simulink model "test_GHV_open_smc"  (R2023b)
settings: Solver=FixedStepAuto  StartTime=0  StopTime=490  FixedStep=0.01  MaxStep=0.001  RelTol=1e-3
InitFcn:
  | run("init.m");
  | %load('feature_point_control_parameters.mat','feature_point_control_parameters');
model workspace (MAT data in the model file):
  initPosLLA = [0; 0; 30000]
undefined symbols (not defined in the file or in its folder): alpha_d_sample, GHV_cfg, t_sample
libraries: simulink_extras x6, aerolibasang x3, aerolibtransform2 x2, aerolib6dof2 x1, aerolibatmos2 x1, matrix_library x1, aerolibgravity2 x1, rllib x1
settings Model: SimulationMode=accelerator  Creator=Admin  LastModifiedBy=Admin
settings SolverCC: AllowMultiTaskInputOutput=on  ZeroCrossControl=EnableAll  ZeroCrossAlgorithm=Adaptive  AutoInsertRateTranBlk=on
settings DataIOCC: Refine=5
settings DebuggingCC: IgnoredZcDiagnostic=none

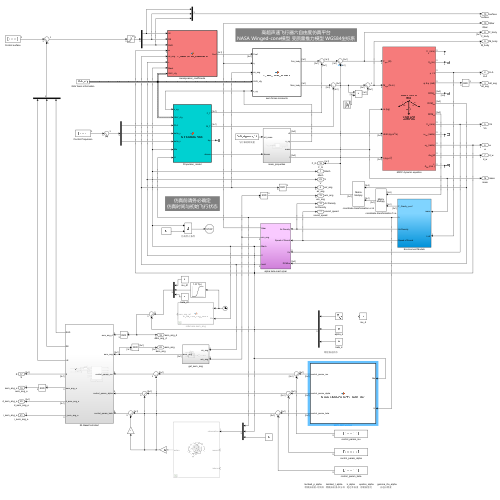
[thumbnail: Simulink's stored preview of the top-level diagram]
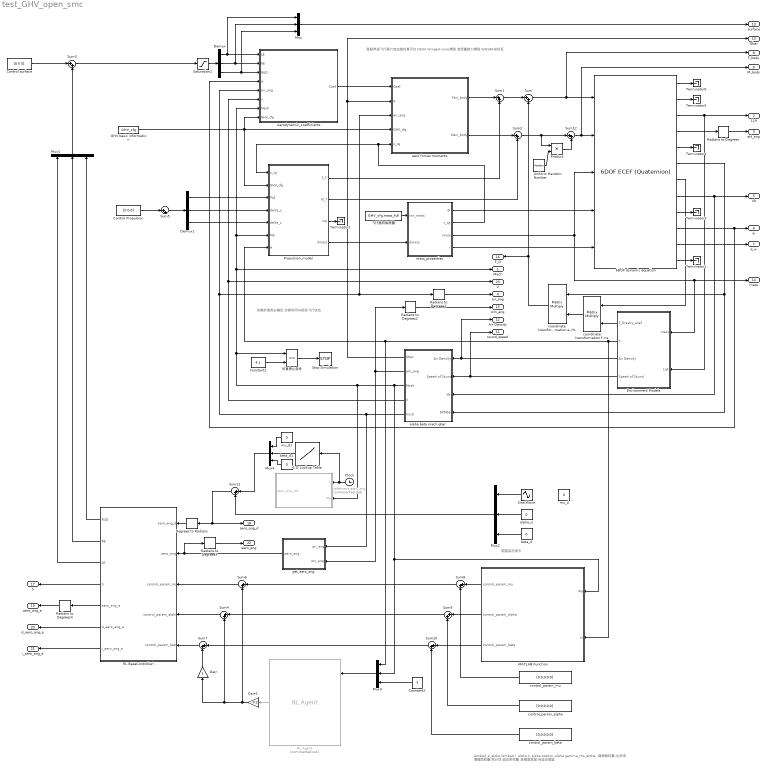
== system test_GHV_open_smc ==
  note: lambad_p_alpha       lambad_I_alpha       k_alpha       epsilon_alpha      gamma_rho_alpha
      | 增模面权重-比例项   增模面权重-积分项   趋近率权重   滑模面宽度             自适应增蓝
  note: 高超声速飞行器六自由度仿真平台
      | NASA Winged-cone模型 变质量推力模型 WGS84坐标系
  note: 仿真前请务必确定
      | 仿真时间与初始飞行状态
  note: 期望姿态指令
  1-D Lookup Table : Lookup_n-D  NumberOfTableDimensions=1  BreakpointsForDimension1=t_sample  Table=alpha_d_sample  InternalRulePriority=Speed  RndMeth=Simplest
  6DOF dynamic equation : aerolib6dof2/6DOF ECEF (Quaternion)  units=Metric (MKS)  mtype=Custom Variable  xg_0=LLA_init  Vm_0=Speed_init  eul_0=Euler_init  pm_0=Omega_init  mass_0=1.0  mass_e=0.5  mass_f=2.0  inertia=eye(3)  inertia_e=eye(3)  inertia_f=2*eye(3)  vre_flag=off  abi_flag=off  ptype=Custom  R=6378137  F=1/298.257223563  w_E=0  angle_in=Internal  LPM0=0  quat_statename=''  pm_statename=''  Vm_statename=''  posfixedframe_statename=''  posinertial_statename=''  LPM_statename=''  mass_statename=''
      settings: LibrarySourceBlock=|
      | aerolib6dof2/Custom Variable Mass 6DOF
      | ECEF (Quaternion)
  Aerodynamic_coefficients : MATLAB Function  TreatAsAtomicUnit=on
  Clock : Clock
  Constant1 : Constant  Value=4.1
  Constant2 : Constant  Value=5
  Control Propulsion : Constant  Value=[0 0 0]
  Control surface : Constant  Value=[0 0 0]
  Degrees to Radians : simulink_extras/Transformations/Degrees to Radians
  Demux : Demux  Outputs=3
  Demux1 : Demux  Outputs=3
  Environment Models : Subsystem
  GHV basic information : Constant  Value=GHV_cfg  VectorParams1D=off  OutDataTypeStr=Bus: slBus1
  Gain : Gain
  Gain1 : Gain  Gain=-0.2
  MATLAB Function : MATLAB Function  TreatAsAtomicUnit=on
  Mux{,1..4} (5 alike) : Mux  Inputs=3
  Product : Product
  Propulsion_model : MATLAB Function  TreatAsAtomicUnit=on
  RL Agent : rllib/RL Agent  Commented=on  Agent=agent_smc_RL_Trained_1  ExternalActionAsInput=off  ProvideLastAction=off  ProvideCumRwd=off  TreatAsDirectFeedthrough=on  UseStrictObservationDataTypes=off
  RL BaseControllerl : Subsystem
  Radians to Degrees{,1..4} (5 alike) : simulink_extras/Transformations/Radians to Degrees
  Saturation1 : Saturate  UpperLimit=30  LowerLimit=-30  ZeroCross=off
  Sine Wave : Sin  Amplitude=30  Frequency=0.05  SampleTime=0
  Stop Simulation : Stop
  Sum{,1..12} (13 alike) : Sum  Inputs=|++
  Terminator{1..6} (6 alike) : Terminator
  Uniform Random Number : UniformRandomNumber  Minimum=-0.1  Maximum=0.1  Seed=42  SampleTime=0.01
  aero forces moments : MATLAB Function  TreatAsAtomicUnit=on
  alpha beta mach qbar : Subsystem
  alpha_d : Constant  Value=0
  beta_d : Constant  Value=0
  beta_d1 : Constant  Value=0
  control_param_alpha : Constant  Value=[0;0;0;0;0]
  control_param_beta : Constant  Value=[0;0;0;0;0]
  control_param_mu : Constant  Value=[0;0;0;0;0]
  coordinate transformation e->b : Product  Multiplication=Matrix(*)
  coordinate transformation f->e : Product  Multiplication=Matrix(*)
  get_aero_ang : Subsystem
  mass_properties : Subsystem
  mu_d : Constant  Value=0
  mu_d1 : Constant  Value=0
  refernece aero_ang : MATLAB Function  Commented=on  TreatAsAtomicUnit=on
  仿真停止条件 : RelationalOperator  Operator=<=  OutDataTypeStr=boolean  RndMeth=Simplest  InputSameDT=off
  飞行器初始质量 : Constant  Value=GHV_cfg.mass_full
  Mach : Outport  SignalName=Mach
  LLA : Outport  Port=2  SignalName=LLA
  att_ang : Outport  Port=3  SignalName=att_ang
  air_ang : Outport  Port=4  SignalName=air_ang
  Vb : Outport  Port=5  SignalName=Vb
  w : Outport  Port=6  SignalName=w
  d_w : Outport  Port=7  SignalName=d_w
  F_body : Outport  Port=8  SignalName=F_body
  M_body : Outport  Port=9  SignalName=M_body
  Qbar : Outport  Port=10  SignalName=Qbar
  sound_speed : Outport  Port=11  SignalName=sound_speed
  Air Density : Outport  Port=12  SignalName=Air Density
  surface : Outport  Port=13  SignalName=surface
  mass : Outport  Port=14  SignalName=mass
  win_ang : Outport  Port=15  SignalName=win_ang
  F_G : Outport  Port=16  SignalName=F_G
  S : Outport  Port=17  SignalName=S
  aero_ang_d : Outport  Port=18  SignalName=aero_ang_d
  aero_ang_e : Outport  Port=19  SignalName=aero_ang_e
  d_aero_ang_e : Outport  Port=20  SignalName=d_aero_ang_e
  i_aero_ang_e : Outport  Port=21  SignalName=i_aero_ang_e
  aero_ang : Outport  Port=22  SignalName=aero_ang
  V : Outport  Port=23  SignalName=V
  wires:
  Control surface/1 -> Sum3/1
  coordinate transformation e->b/1 -> Sum/2, F_G/1
  Aerodynamic_coefficients/1(Coef) -> aero forces moments/1(Coef)
  mass_properties/2(x_cg) -> aero forces moments/5(x_cg), Propulsion_model/1(x_cg)
  coordinate transformation f->e/1 -> coordinate transformation e->b/2
  飞行器初始质量/1 -> mass_properties/1(init_mass)
  Radians to Degrees1/1 -> air_ang/1
  Propulsion_model/2(M_T) -> Sum2/2
  6DOF dynamic equation/1 -> Terminator6/1
  6DOF dynamic equation/9 -> Terminator3/1
  mass_properties/3(mass) -> 6DOF dynamic equation/3, Environment Models/1(mass), mass/1
  Radians to Degrees2/1 -> win_ang/1
  Demux/1 -> Aerodynamic_coefficients/1(LE), Mux/1
  6DOF dynamic equation/5 -> Terminator4/1
  Saturation1/1 -> Demux/1
  Demux1/2 -> Propulsion_model/4(delta_y)
  Control Propulsion/1 -> Sum5/1
  Propulsion_model/1(F_T) -> Sum1/2
  Demux/2 -> Aerodynamic_coefficients/2(RE), Mux/2
  alpha beta mach qbar/5(Incid) -> Aerodynamic_coefficients/5(air_ang), aero forces moments/3(air_ang), Radians to Degrees1/1, get_aero_ang/1(air_ang)
  Sum2/1 -> Sum12/1, Product/1
  Propulsion_model/4(dmass) -> mass_properties/2(dmass)
  Sum1/1 -> Sum/1
  Environment Models/3(Air Density) -> Air Density/1, alpha beta mach qbar/1(Air Density)
  Environment Models/2(h) -> Propulsion_model/7(H), Mux3/1, MATLAB Function/2(H)
  alpha beta mach qbar/1(Qbar) -> aero forces moments/2(q), Qbar/1
  aero forces moments/1(Fair_body) -> Sum1/1
  Radians to Degrees/1 -> att_ang/1
  aero forces moments/2(Mair_body) -> Sum2/1
  Demux1/3 -> Propulsion_model/5(delta_z)
  6DOF dynamic equation/10 -> w/1, Aerodynamic_coefficients/4(w)
  Mux/1 -> surface/1
  GHV basic information/1 -> aero forces moments/4(GHV_cfg), Propulsion_model/2(GHV_cfg), Aerodynamic_coefficients/8(GHV_cfg)
  Demux/3 -> Aerodynamic_coefficients/3(RUD), Mux/3
  alpha beta mach qbar/2(win_ang) -> Radians to Degrees2/1, get_aero_ang/2(win_ang)
  Sum3/1 -> Saturation1/1
  Propulsion_model/3(Isp) -> Terminator2/1
  Environment Models/1(F_Gravity_ecef) -> coordinate transformation f->e/2
  6DOF dynamic equation/11 -> d_w/1
  Demux1/1 -> Propulsion_model/3(PLA)
  mass_properties/1(dI) -> 6DOF dynamic equation/4
  6DOF dynamic equation/7 -> coordinate transformation f->e/1
  6DOF dynamic equation/2 -> Terminator5/1
  6DOF dynamic equation/8 -> Vb/1, alpha beta mach qbar/3(Vb)
  alpha beta mach qbar/4(V) -> Aerodynamic_coefficients/6(v), V/1
  Environment Models/4(Speed of Sound) -> sound_speed/1, alpha beta mach qbar/2(Speed of Sound)
  6DOF dynamic equation/12 -> Terminator1/1
  6DOF dynamic equation/4 -> Radians to Degrees/1
  Sum/1 -> 6DOF dynamic equation/1, F_body/1
  mass_properties/4(I) -> 6DOF dynamic equation/5
  Sum5/1 -> Demux1/1
  alpha beta mach qbar/3(Mach) -> Aerodynamic_coefficients/7(Mach), Propulsion_model/6(Ma), Mach/1, 仿真停止条件/1, refernece aero_ang/2(Ma), MATLAB Function/1(Ma), Mux3/2
  Constant1/1 -> 仿真停止条件/2
  仿真停止条件/1 -> Stop Simulation/1
  get_aero_ang/1(aero_ang) -> Radians to Degrees3/1, RL BaseControllerl/2(aero_ang)
  Sum11/1 -> Degrees to Radians/1, aero_ang_d/1
  RL BaseControllerl/1(RUD) -> Mux1/3
  RL BaseControllerl/2(RE) -> Mux1/2
  RL BaseControllerl/3(LE) -> Mux1/1
  RL BaseControllerl/4(S) -> S/1
  Degrees to Radians/1 -> RL BaseControllerl/1(aero_ang_d)
  Mux1/1 -> Sum3/2
  RL BaseControllerl/5(aero_ang_e) -> Radians to Degrees4/1
  RL BaseControllerl/6(d_aero_ang_e) -> d_aero_ang_e/1
  RL BaseControllerl/7(i_aero_ang_e) -> i_aero_ang_e/1
  6DOF dynamic equation/6 -> alpha beta mach qbar/4(DCMbe), coordinate transformation e->b/1
  6DOF dynamic equation/3 -> LLA/1, Environment Models/2(LLA)
  Sum6/1 -> RL BaseControllerl/3(control_param_mu)
  Radians to Degrees3/1 -> aero_ang/1
  Sum4/1 -> RL BaseControllerl/4(control_param_alpha)
  beta_d/1 -> Mux2/3
  alpha_d/1 -> Mux2/2
  Radians to Degrees4/1 -> aero_ang_e/1
  Mux3/1 -> RL Agent/1
  Constant2/1 -> Mux3/3
  Sum9/1 -> Sum4/1
  Sum8/1 -> Sum6/1
  RL Agent/1 -> Gain1/1
  Sum10/1 -> Sum7/1
  Gain/1 -> Sum7/2
  MATLAB Function/1(control_param_mu) -> Sum8/1
  MATLAB Function/2(control_param_alpha) -> Sum9/1
  MATLAB Function/3(control_param_beta) -> Sum10/1
  control_param_mu/1 -> Sum8/2
  control_param_alpha/1 -> Sum9/2
  control_param_beta/1 -> Sum10/2
  Clock/1 -> 1-D Lookup Table/1, refernece aero_ang/1(t)
  Mux2/1 -> Sum11/2
  Sum7/1 -> RL BaseControllerl/5(control_param_bate)
  Sine Wave/1 -> Mux2/1
  Gain1/1 -> Gain/1, Sum4/2, Sum6/2
  1-D Lookup Table/1 -> Mux4/2
  Mux4/1 -> Sum11/1
  mu_d1/1 -> Mux4/1
  beta_d1/1 -> Mux4/3
  Uniform Random Number/1 -> Product/2
  Sum12/1 -> M_body/1, 6DOF dynamic equation/2
  Product/1 -> Sum12/2

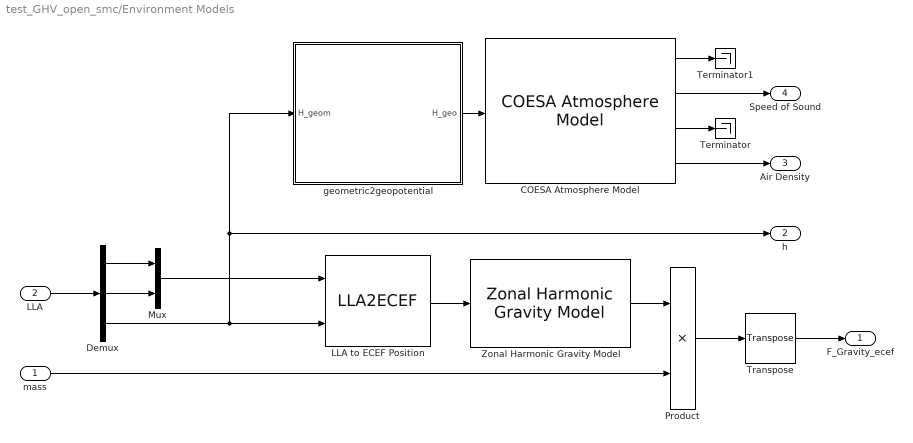
== system test_GHV_open_smc/Environment Models ==
  mass : Inport
  LLA : Inport  Port=2
  COESA Atmosphere Model : aerolibatmos2/COESA Atmosphere Model  units=Metric (MKS)  spec=1976 COESA-extended U.S. Standard Atmosphere  model=Profile  profile_var=High temperature  profile_percent=1%  profile_alt=5 km (16404 ft)  envelope_var=High temperature  envelope_percent=1%  action=Warning
  Demux : Demux  Outputs=3
  LLA to ECEF Position : LLA2ECEF
  Mux : Mux  Inputs=2
  Product : Product
  Terminator : Terminator
  Terminator1 : Terminator
  Transpose : matrix_library/Transpose
  Zonal Harmonic Gravity Model : aerolibgravity2/Zonal Harmonic Gravity Model  units=Metric (MKS)  degree=2  action=Warning  ptype=Earth  R=6378136.3  GM=398600441500000  jvalue=[1.0826269e-03 -2.5323000e-06 -1.6204000e-06]
  geometric2geopotential : MATLAB Function  TreatAsAtomicUnit=on
  F_Gravity_ecef : Outport
  h : Outport  Port=2
  Air Density : Outport  Port=3
  Speed of Sound : Outport  Port=4
  wires:
  COESA Atmosphere Model/1 -> Terminator1/1
  COESA Atmosphere Model/2 -> Speed of Sound/1
  COESA Atmosphere Model/3 -> Terminator/1
  COESA Atmosphere Model/4 -> Air Density/1
  LLA to ECEF Position/1 -> Zonal Harmonic Gravity Model/1
  Mux/1 -> LLA to ECEF Position/1
  Demux/3 -> h/1, geometric2geopotential/1(H_geom), LLA to ECEF Position/2
  Demux/1 -> Mux/1
  Demux/2 -> Mux/2
  LLA/1 -> Demux/1
  mass/1 -> Product/2
  Zonal Harmonic Gravity Model/1 -> Product/1
  Product/1 -> Transpose/1
  Transpose/1 -> F_Gravity_ecef/1
  geometric2geopotential/1(H_geo) -> COESA Atmosphere Model/1

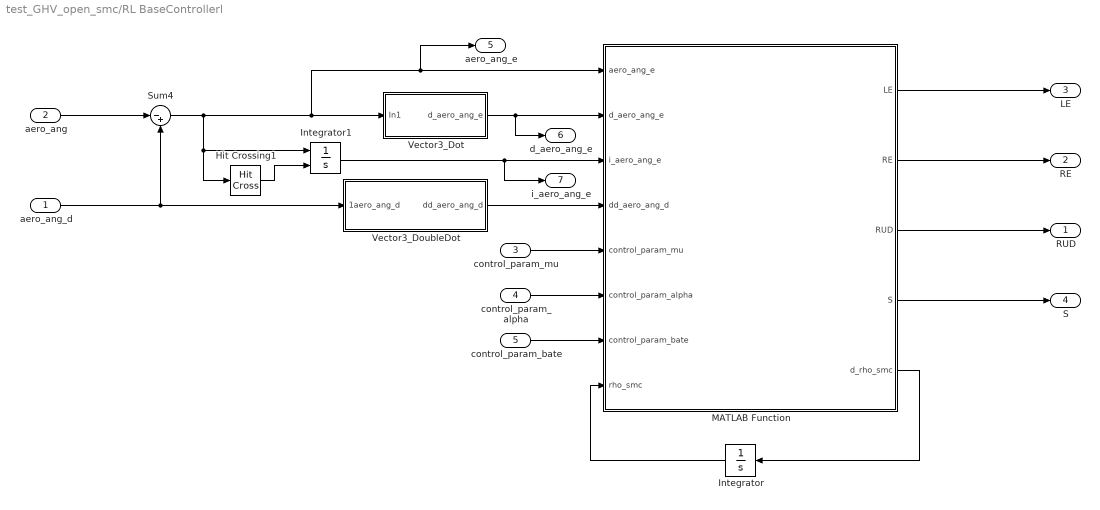
== system test_GHV_open_smc/RL BaseControllerl ==
  aero_ang_d : Inport
  aero_ang : Inport  Port=2
  control_param_mu : Inport  Port=3
  control_param_alpha : Inport  Port=4
  control_param_bate : Inport  Port=5
  Hit Crossing1 : HitCross
  Integrator : Integrator  InitialCondition=[0;10;0]
  Integrator1 : Integrator  ExternalReset=either
  MATLAB Function : MATLAB Function  TreatAsAtomicUnit=on
  Sum4 : Sum  Inputs=|-+
  Vector3_Dot : Subsystem
  Vector3_DoubleDot : Subsystem
  RUD : Outport
  RE : Outport  Port=2
  LE : Outport  Port=3
  S : Outport  Port=4
  aero_ang_e : Outport  Port=5
  d_aero_ang_e : Outport  Port=6
  i_aero_ang_e : Outport  Port=7
  wires:
  control_param_alpha/1 -> MATLAB Function/6(control_param_alpha)
  Vector3_DoubleDot/1(dd_aero_ang_d) -> MATLAB Function/4(dd_aero_ang_d)
  MATLAB Function/5(d_rho_smc) -> Integrator/1
  MATLAB Function/2(RE) -> RE/1
  aero_ang_d/1 -> Sum4/2, Vector3_DoubleDot/1(1aero_ang_d)
  MATLAB Function/1(LE) -> LE/1
  Integrator1/1 -> MATLAB Function/3(i_aero_ang_e), i_aero_ang_e/1
  MATLAB Function/3(RUD) -> RUD/1
  MATLAB Function/4(S) -> S/1
  Integrator/1 -> MATLAB Function/8(rho_smc)
  Sum4/1 -> Hit Crossing1/1, Integrator1/1, aero_ang_e/1, MATLAB Function/1(aero_ang_e), Vector3_Dot/1(In1)
  aero_ang/1 -> Sum4/1
  Hit Crossing1/1 -> Integrator1/2
  Vector3_Dot/1(d_aero_ang_e) -> MATLAB Function/2(d_aero_ang_e), d_aero_ang_e/1
  control_param_bate/1 -> MATLAB Function/7(control_param_bate)
  control_param_mu/1 -> MATLAB Function/5(control_param_mu)

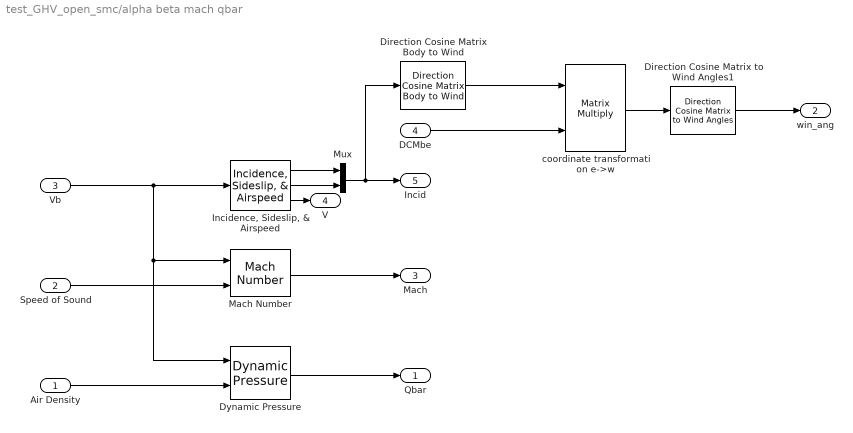
== system test_GHV_open_smc/alpha beta mach qbar ==
  Air Density : Inport
  Speed of Sound : Inport  Port=2
  Vb : Inport  Port=3
  DCMbe : Inport  Port=4
  Direction Cosine Matrix Body to Wind : aerolibtransform2/Direction Cosine Matrix Body to Wind
  Direction Cosine Matrix to Wind Angles1 : aerolibtransform2/Direction Cosine Matrix to Wind Angles  action=None  tolerance=eps(2)
  Dynamic Pressure : aerolibasang/Dynamic Pressure
  "Incidence, Sideslip, & Airspeed" : aerolibasang/Incidence, Sideslip, & Airspeed
  Mach Number : aerolibasang/Mach Number
  Mux : Mux  Inputs=2
  coordinate transformation e->w : Product  Multiplication=Matrix(*)
  Qbar : Outport
  win_ang : Outport  Port=2
  Mach : Outport  Port=3
  V : Outport  Port=4
  Incid : Outport  Port=5
  wires:
  Speed of Sound/1 -> Mach Number/2
  Mach Number/1 -> Mach/1
  "Incidence, Sideslip, & Airspeed"/2 -> Mux/2
  Vb/1 -> Dynamic Pressure/1, Mach Number/1, "Incidence, Sideslip, & Airspeed"/1
  Dynamic Pressure/1 -> Qbar/1
  Mux/1 -> Direction Cosine Matrix Body to Wind/1, Incid/1
  "Incidence, Sideslip, & Airspeed"/1 -> Mux/1
  Air Density/1 -> Dynamic Pressure/2
  "Incidence, Sideslip, & Airspeed"/3 -> V/1
  DCMbe/1 -> coordinate transformation e->w/2
  Direction Cosine Matrix Body to Wind/1 -> coordinate transformation e->w/1
  coordinate transformation e->w/1 -> Direction Cosine Matrix to Wind Angles1/1
  Direction Cosine Matrix to Wind Angles1/1 -> win_ang/1

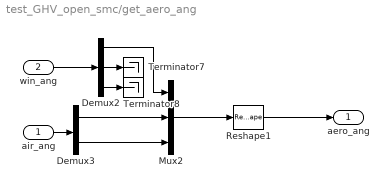
== system test_GHV_open_smc/get_aero_ang ==
  air_ang : Inport
  win_ang : Inport  Port=2
  Demux2 : Demux  Outputs=3
  Demux3 : Demux  Outputs=2
  Mux2 : Mux  Inputs=3
  Reshape1 : Reshape  OutputDimensionality=Column vector (2-D)
  Terminator7 : Terminator
  Terminator8 : Terminator
  aero_ang : Outport
  wires:
  Mux2/1 -> Reshape1/1
  Demux2/2 -> Terminator7/1
  Reshape1/1 -> aero_ang/1
  air_ang/1 -> Demux3/1
  Demux3/1 -> Mux2/2
  win_ang/1 -> Demux2/1
  Demux2/3 -> Terminator8/1
  Demux3/2 -> Mux2/3
  Demux2/1 -> Mux2/1

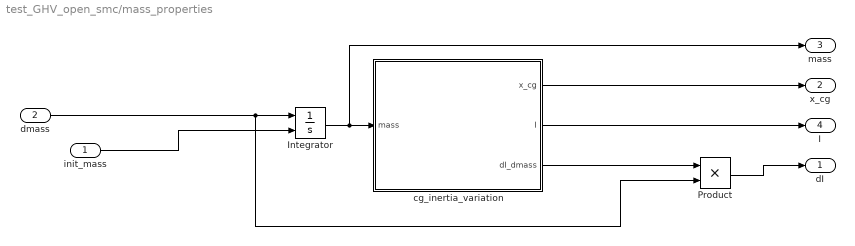
== system test_GHV_open_smc/mass_properties ==
  init_mass : Inport
  dmass : Inport  Port=2
  Integrator : Integrator  InitialConditionSource=external
  Product : Product
  cg_inertia_variation : MATLAB Function  TreatAsAtomicUnit=on
  dI : Outport
  x_cg : Outport  Port=2
  mass : Outport  Port=3
  I : Outport  Port=4
  wires:
  Integrator/1 -> mass/1, cg_inertia_variation/1(mass)
  init_mass/1 -> Integrator/2
  cg_inertia_variation/3(dI_dmass) -> Product/1
  dmass/1 -> Product/2, Integrator/1
  cg_inertia_variation/2(I) -> I/1
  cg_inertia_variation/1(x_cg) -> x_cg/1
  Product/1 -> dI/1

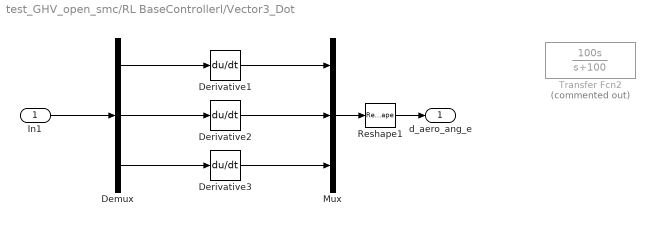
== system test_GHV_open_smc/RL BaseControllerl/Vector3_Dot ==
  In1 : Inport
  Demux : Demux  Outputs=3
  Derivative1 : Derivative
  Derivative2 : Derivative
  Derivative3 : Derivative
  Mux : Mux  Inputs=3
  Reshape1 : Reshape  OutputDimensionality=Column vector (2-D)
  Transfer Fcn2 : TransferFcn  Commented=on  Numerator=[100 0]  Denominator=[1 100]
  d_aero_ang_e : Outport
  wires:
  In1/1 -> Demux/1
  Demux/2 -> Derivative2/1
  Demux/1 -> Derivative1/1
  Demux/3 -> Derivative3/1
  Mux/1 -> Reshape1/1
  Reshape1/1 -> d_aero_ang_e/1
  Derivative1/1 -> Mux/1
  Derivative2/1 -> Mux/2
  Derivative3/1 -> Mux/3

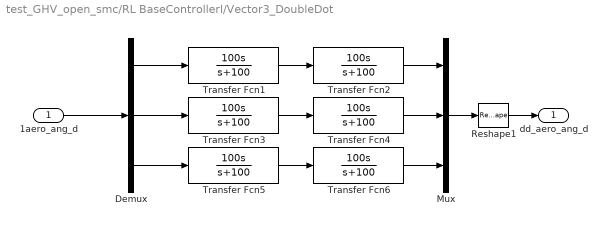
== system test_GHV_open_smc/RL BaseControllerl/Vector3_DoubleDot ==
  1aero_ang_d : Inport
  Demux : Demux  Outputs=3
  Mux : Mux  Inputs=3
  Reshape1 : Reshape  OutputDimensionality=Column vector (2-D)
  Transfer Fcn{1..6} (6 alike) : TransferFcn  Numerator=[100 0]  Denominator=[1 100]
  dd_aero_ang_d : Outport
  wires:
  Transfer Fcn1/1 -> Transfer Fcn2/1
  1aero_ang_d/1 -> Demux/1
  Transfer Fcn3/1 -> Transfer Fcn4/1
  Transfer Fcn5/1 -> Transfer Fcn6/1
  Demux/2 -> Transfer Fcn3/1
  Demux/1 -> Transfer Fcn1/1
  Demux/3 -> Transfer Fcn5/1
  Transfer Fcn4/1 -> Mux/2
  Transfer Fcn6/1 -> Mux/3
  Transfer Fcn2/1 -> Mux/1
  Mux/1 -> Reshape1/1
  Reshape1/1 -> dd_aero_ang_d/1

== matlab function test_GHV_open_smc/MATLAB Function ==
  data: Ma input; H input; control_param_mu output; control_param_alpha output; control_param_beta output
function [control_param_mu, control_param_alpha, control_param_beta] = S_gain_scheduling_control_param_6dof(Ma, H)
control_param_mu =zeros(5,1);
control_param_alpha = zeros(5,1);
control_param_beta = zeros(5,1);
[control_param_mu, control_param_alpha, control_param_beta] = gain_scheduling_control_param_6dof(H, Ma);

end

== matlab function test_GHV_open_smc/Propulsion_model ==
  data: F_T output; M_T output; x_cg input; GHV_cfg input; PLA input; delta_y input; delta_z input; Ma input; H input; Isp output; dmass output
function [F_T,M_T, Isp,  dmass] = S_Propulsion_model(x_cg, GHV_cfg, PLA, delta_y, delta_z, Ma, H)
    F_T = zeros(3, 1); %#ok<PREALL>
    M_T = zeros(3, 1); %#ok<PREALL>
   [F_T, M_T, Isp, dmass] = Propulsion_model(PLA, H, Ma, delta_y, delta_z, GHV_cfg, x_cg);

end

== matlab function test_GHV_open_smc/Aerodynamic_coefficients ==
  data: LE input; Coef output; RE input; RUD input; w input; air_ang input; v input; Mach input; GHV_cfg input
function Coef = S_Aerodynamic_coefficients(LE, RE, RUD, w, air_ang,v, Mach, GHV_cfg)
    Coef = zeros(6, 1);
    Coef = Aerodynamic_coefficients(LE, RE, RUD, air_ang, v, w, Mach, GHV_cfg);
    Coef = [1;1;1;1.2;1.2;1.2].*Coef;

end

== matlab function test_GHV_open_smc/aero forces moments ==
  data: Coef input; q input; air_ang input; GHV_cfg input; x_cg input; Fair_body output; Mair_body output
function [Fair_body, Mair_body] = S_aero_forces_moments(Coef, q, air_ang, GHV_cfg, x_cg)

    Fair_body = zeros(3, 1); %#ok<PREALL>
    Mair_body = zeros(3, 1); %#ok<PREALL>
    [Fair_body, Mair_body] = aero_forces_moments(Coef, q, GHV_cfg, x_cg, air_ang);

end

== matlab function test_GHV_open_smc/Environment Models/geometric2geopotential ==
  data: H_geom input; H_geo output
function H_geo = S_geometric2geopotential(H_geom)

    H_geo = geometric2geopotential(H_geom);

end

== matlab function test_GHV_open_smc/RL BaseControllerl/MATLAB Function ==
  data: aero_ang_e input; d_aero_ang_e input; i_aero_ang_e input; dd_aero_ang_d input; control_param_mu input; LE output; control_param_alpha input; control_param_bate input; rho_smc input; RE output; RUD output; S output; d_rho_smc output
function [LE, RE, RUD, S, d_rho_smc] = S_RL_BaseController(aero_ang_e, d_aero_ang_e, i_aero_ang_e, dd_aero_ang_d, control_param_mu, control_param_alpha, control_param_bate, rho_smc)

[LE, RE, RUD, d_rho_smc, S] = RL_BaseController(dd_aero_ang_d, aero_ang_e, d_aero_ang_e, i_aero_ang_e, rho_smc, control_param_alpha, control_param_bate, control_param_mu);

end

== matlab function test_GHV_open_smc/mass_properties/cg_inertia_variation ==
  data: mass input; x_cg output; I output; dI_dmass output
function [x_cg, I, dI_dmass] = S_cg_inertia_variation(mass)

     [x_cg, I, dI_dmass] = cg_inertia_variation(mass);
     
end

== matlab function test_GHV_open_smc/refernece aero_ang ==
  data: t input; Ma input; aero_ang_ref output
function aero_ang_ref = S_ref_aero_ang_dDOF(t, Ma)

    aero_ang_ref = ref_aero_ang_dDOF(t, Ma);

end
